simulink model "Simulink_progetto_lineare"  (R2023b)
settings: Solver=VariableStepAuto  StartTime=0.0  StopTime=0.02  RelTol=1e-3
libraries: cstblocks x2
settings Model: Creator=guidocarnevale  LastModifiedBy=aleor

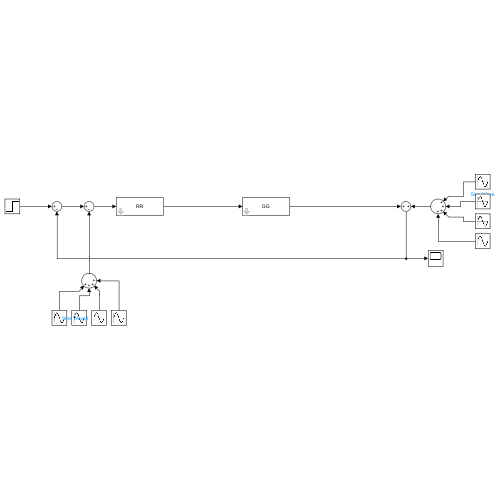
[thumbnail: Simulink's stored preview of the top-level diagram]
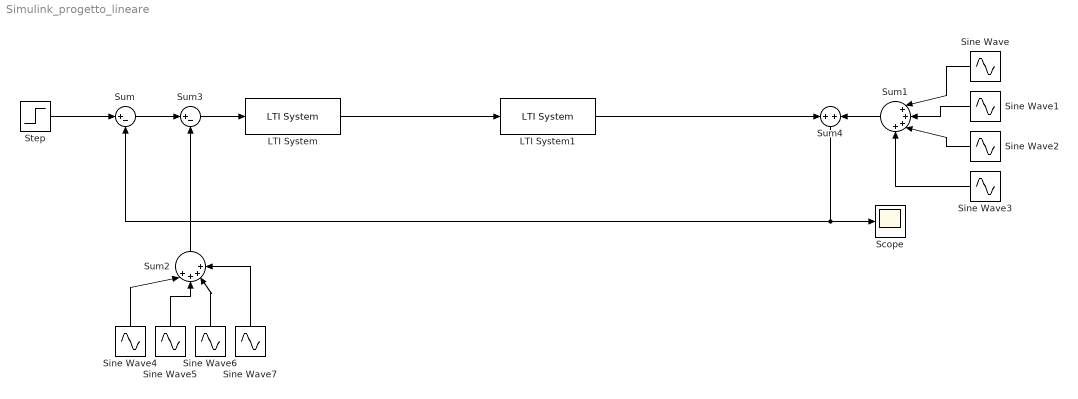
== system Simulink_progetto_lineare ==
  LTI System : cstblocks/LTI System  Tag=R  sys=RR  IC=[]  PadeOrder=0
  LTI System1 : cstblocks/LTI System  Tag=R  sys=GG  IC=[]  PadeOrder=0
  Scope : Scope
  Sine Wave : Sin  Amplitude=10  Frequency=0.15  SampleTime=0
  Sine Wave1 : Sin  Amplitude=10  Frequency=0.30  SampleTime=0
  Sine Wave2 : Sin  Amplitude=10  Frequency=0.45  SampleTime=0
  Sine Wave3 : Sin  Amplitude=10  Frequency=0.60  SampleTime=0
  Sine Wave4 : Sin  Frequency=100000  SampleTime=0
  Sine Wave5 : Sin  Frequency=200000  SampleTime=0
  Sine Wave6 : Sin  Frequency=300000  SampleTime=0
  Sine Wave7 : Sin  Frequency=400000  SampleTime=0
  Step : Step  Time=0  SampleTime=0
  Sum : Sum  Inputs=|+-
  Sum1 : Sum  Inputs=|++++
  Sum2 : Sum  Inputs=|++++
  Sum3 : Sum  Inputs=|+-
  Sum4 : Sum  Inputs=+|+
  wires:
  Sum/1 -> Sum3/1
  LTI System/1 -> LTI System1/1
  Sum3/1 -> LTI System/1
  Sum1/1 -> Sum4/2
  LTI System1/1 -> Sum4/1
  Sum4/1 -> Sum/2, Scope/1
  Step/1 -> Sum/1
  Sine Wave/1 -> Sum1/1
  Sine Wave1/1 -> Sum1/2
  Sine Wave2/1 -> Sum1/3
  Sine Wave3/1 -> Sum1/4
  Sine Wave4/1 -> Sum2/1
  Sine Wave6/1 -> Sum2/3
  Sine Wave5/1 -> Sum2/2
  Sine Wave7/1 -> Sum2/4
  Sum2/1 -> Sum3/2
